simulink model "RR_grasping"  (R2020b)
settings: Solver=FixedStepAuto  StartTime=0  StopTime=10.0  FixedStep=0.001  MaxStep=0.05  RelTol=1e-3
values from neighbouring files (symbols this model uses):
  a0 = 0.99    [init.m]
  berta = 0.98    [init.m]
  csi = 1    [init.m]
  e_max = 0.05    [init.m]
  F_max = [2;2]    [init.m]
  F_weight = [0;-50]    [init.m]
  g = 9.81    [init.m]
  I1 = 1    [init.m]
  I2 = 1    [init.m]
  l1 = 1    [init.m]
  l2 = 1    [init.m]
  m1 = 1    [init.m]
  m2 = 1    [init.m]
  mass = 1    [init.m]
libraries: cstblocks x2, simulink x1
settings Model: Creator=chiara-s  LastModifiedBy=chiara-s

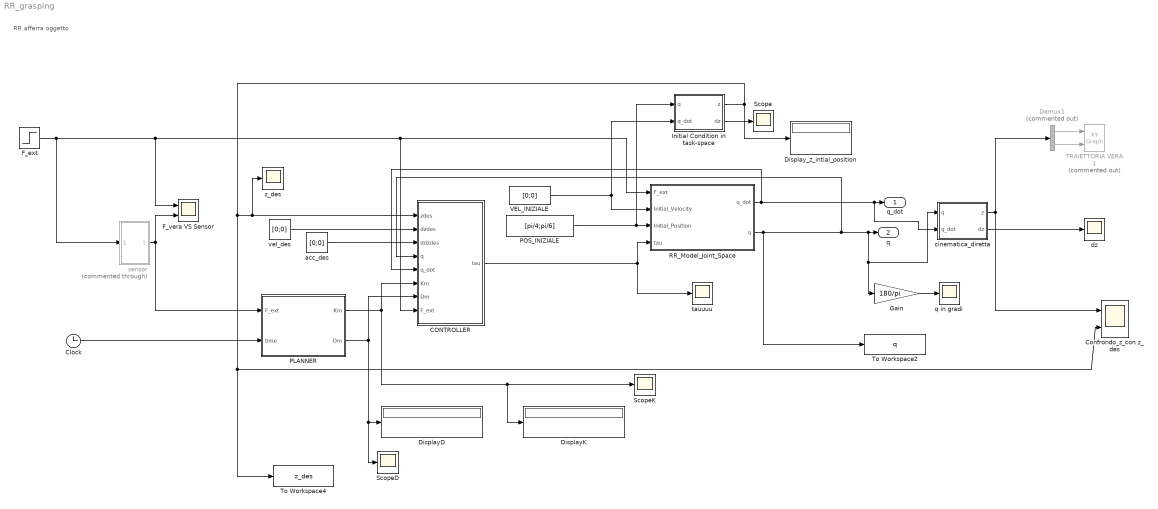
== system RR_grasping ==
  note: RR afferra oggetto
  CONTROLLER : MATLAB Function  TreatAsAtomicUnit=on
  Clock : Clock
  Confrondo_z_con z_des : Scope  NumInputPorts=2
  Demux1 : Demux  Commented=on  Outputs=2
  DisplayD : Display
  DisplayK : Display
  Display_z_intial_position : Display
  F_ext : Step  Before=[0;0]  After=2*F_weight  SampleTime=0
  F_vera VS Sensor : Scope  NumInputPorts=2
  Gain : Gain  Gain=180/pi
  Initial Condition in task-space : MATLAB Function  TreatAsAtomicUnit=on
  PLANNER : MATLAB Function  TreatAsAtomicUnit=on
  POS_INIZIALE : Constant  Value=[pi/4;pi/6]
  RR_Model_Joint_Space : Subsystem
  Scope : Scope
  ScopeD : Scope
  ScopeK : Scope
  TRAIETTORIA VERA 1 : simulink/Sinks/XY Graph  Commented=on  xmin=-2  xmax=2  ymin=-2  ymax=2  st=-1
  To Workspace2 : ToWorkspace  VariableName=q  SaveFormat=Structure With Time  SampleTime=-1
      settings: Save2DSignal=2-D array (concatenate along first dimension)
  To Workspace4 : ToWorkspace  VariableName=z_des  SaveFormat=Structure With Time  SampleTime=-1
      settings: Save2DSignal=2-D array (concatenate along first dimension)
  VEL_INIZIALE : Constant  Value=[0;0]
  acc_des : Constant  Value=[0;0]
  cinematica_diretta : MATLAB Function  TreatAsAtomicUnit=on
  dz : Scope
  q in gradi : Scope
  sensor : Subsystem  Commented=through
  tauuuu : Scope
  vel_des : Constant  Value=[0;0]
  z_des : Scope
  q_dot : Outport
  q : Outport  Port=2
  wires:
  RR_Model_Joint_Space/1(q_dot) -> cinematica_diretta/2(q_dot), q_dot/1, CONTROLLER/5(q_dot)
  Initial Condition in task-space/1(z) -> z_des/1, CONTROLLER/1(zdes), To Workspace4/1, Confrondo_z_con z_des/2, Display_z_intial_position/1
  F_ext/1 -> sensor/1(In1), RR_Model_Joint_Space/1(F_ext), CONTROLLER/8(F_ext), F_vera VS Sensor/1
  CONTROLLER/1(tau) -> tauuuu/1, RR_Model_Joint_Space/4(tau)
  PLANNER/1(Km) -> CONTROLLER/6(Km), ScopeK/1, DisplayK/1
  vel_des/1 -> CONTROLLER/2(dzdes)
  Demux1/2 -> TRAIETTORIA VERA 1/2
  PLANNER/2(Dm) -> CONTROLLER/7(Dm), ScopeD/1, DisplayD/1
  RR_Model_Joint_Space/2(q) -> CONTROLLER/4(q), Gain/1, cinematica_diretta/1(q), q/1, To Workspace2/1
  Demux1/1 -> TRAIETTORIA VERA 1/1
  cinematica_diretta/1(z) -> Confrondo_z_con z_des/1, Demux1/1
  cinematica_diretta/2(dz) -> dz/1
  POS_INIZIALE/1 -> RR_Model_Joint_Space/3(Initial_Position), Initial Condition in task-space/1(q)
  Gain/1 -> q in gradi/1
  VEL_INIZIALE/1 -> Initial Condition in task-space/2(q_dot), RR_Model_Joint_Space/2(Initial_Velocity)
  acc_des/1 -> CONTROLLER/3(ddzdes)
  Initial Condition in task-space/2(dz) -> Scope/1
  Clock/1 -> PLANNER/2(time)
  sensor/1(Out1) -> PLANNER/1(F_ext), F_vera VS Sensor/2

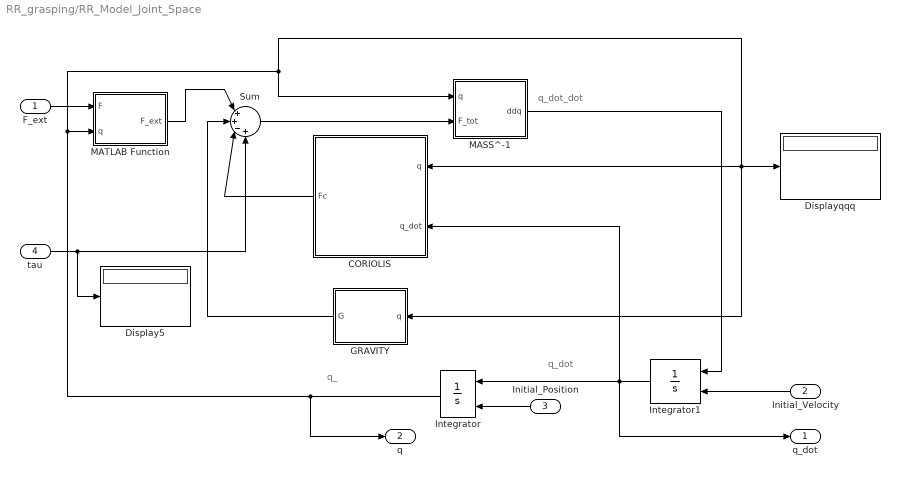
== system RR_grasping/RR_Model_Joint_Space ==
  note: q_dot
  note: q_dot_dot
  note: q_
  F_ext : Inport
  Initial_Velocity : Inport  Port=2
  Initial_Position : Inport  Port=3
  tau : Inport  Port=4
  CORIOLIS : MATLAB Function  TreatAsAtomicUnit=on
  Display5 : Display
  Displayqqq : Display
  GRAVITY : MATLAB Function  TreatAsAtomicUnit=on
  Integrator : Integrator  InitialConditionSource=external
  Integrator1 : Integrator  InitialConditionSource=external  InitialCondition=[0;0]
  MASS^-1 : MATLAB Function  TreatAsAtomicUnit=on
  MATLAB Function : MATLAB Function  TreatAsAtomicUnit=on
  Sum : Sum  Inputs=|++-+
  q_dot : Outport
  q : Outport  Port=2
  wires:
  GRAVITY/1(G) -> Sum/2
  MATLAB Function/1(F_ext) -> Sum/1
  Initial_Position/1 -> Integrator/2
  F_ext/1 -> MATLAB Function/1(F)
  Integrator/1 -> MASS^-1/1(q), GRAVITY/1(q), Displayqqq/1, CORIOLIS/1(q), MATLAB Function/2(q), q/1
  Integrator1/1 -> q_dot/1, CORIOLIS/2(q_dot), Integrator/1
  Initial_Velocity/1 -> Integrator1/2
  MASS^-1/1(ddq) -> Integrator1/1
  Sum/1 -> MASS^-1/2(F_tot)
  CORIOLIS/1(Fc) -> Sum/3
  tau/1 -> Display5/1, Sum/4

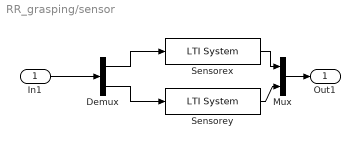
== system RR_grasping/sensor ==
  In1 : Inport
  Demux : Demux  Outputs=2
  Mux : Mux  Inputs=2
  Sensorex : cstblocks/LTI System  sys=tf(50^2,[1 0.3*2*50 50^2])  IC=[]
  Sensorey : cstblocks/LTI System  sys=tf(50^2,[1 0.3*2*50 50^2])  IC=[]
  Out1 : Outport
  wires:
  Demux/1 -> Sensorex/1
  Sensorex/1 -> Mux/1
  Sensorey/1 -> Mux/2
  Mux/1 -> Out1/1
  Demux/2 -> Sensorey/1
  In1/1 -> Demux/1

== matlab function RR_grasping/RR_Model_Joint_Space/MATLAB Function ==
  data: F input size=2; F_ext output double size=2; q input size=2; l1 parameter; l2 parameter
function F_ext = fcn(F,q,l1, l2)


Ja = [-l1*sin(q(1)) - l2*sin(q(1)+q(2)), -l2*sin(q(1)+q(2)); ...
    l1*cos(q(1)) + l2*cos(q(1)+q(2)), l2*cos(q(1)+q(2))];

F_ext = Ja'*F;

end

== matlab function RR_grasping/cinematica_diretta ==
  data: q input double size=2; q_dot input double size=2; z output double size=2; dz output double size=2; l1 parameter; l2 parameter
function [z,dz] = fcn(q,q_dot,l1, l2)

z = zeros(2,1);
z(1) = l1*cos(q(1)) + l2*cos(q(1)+q(2));
z(2) = l1*sin(q(1)) + l2*sin(q(1)+q(2));

Ja = zeros(2,2);
Ja = [-l1*sin(q(1)) - l2*sin(q(1)+q(2)), -l2*sin(q(1)+q(2)); ...
    l1*cos(q(1)) + l2*cos(q(1)+q(2)), l2*cos(q(1)+q(2))];

dz = zeros(2,1);
dz = Ja*q_dot;

end

== matlab function RR_grasping/CONTROLLER ==
  data: zdes input size=2; tau output double size=2; dzdes input size=2; ddzdes input size=2; q input size=2; q_dot input size=2; Km input; Dm input; F_ext input; M parameter
function tau = fcn(zdes, dzdes, ddzdes, q, q_dot, Km, Dm, F_ext, M)
%% PROBLEMA MATRICE DELLE MASSE NON DIAGONALE
coder.extrinsic('Jacobianoa','Jacobianoa_dot','Mass','Coriolis','Gravity','cin_dir')
dz = zeros(2,1);
z = zeros(2,1);
B = zeros(2,2);
S = zeros(2,2);
G = zeros(2,1);
Ja = zeros(2,2);
Ja_dot = zeros(2,2);
Bm = [M 0; 0 M];
Ja = Jacobianoa(q);
Ja_dot = Jacobianoa_dot(q,q_dot);

dz = Ja*q_dot;
z = cin_dir(q);

t = 0.1;
if (deg2rad(-0.1) < q(2)) && (q(2) < deg2rad(0.1)) || (deg2rad(179.9) < q(2)) && (q(2) < deg2rad(180.1)) || (deg2rad(-180.1) < q(2)) && (q(2) < deg2rad(-179.9))
    Ja_inv = (Ja')*inv(Ja*(Ja') + t^2*eye(2,2)); % Damp least square Jacobian method
else 
    Ja_inv = inv(Ja);
end

% Ja_inv = inv(Ja);

B = Mass(q);
Bx = (Ja_inv')* B * Ja_inv;
S = Coriolis(q,q_dot);
G = Gravity(q);
I = eye(2,2);
% tau = B * Ja_inv*(ddzdes - Ja_dot*q_dot) + ...
%     S*q_dot + (Ja')*(Dm*(dzdes - dz) + Km*(zdes- z)) + G;

tau = B*Ja_inv*(ddzdes - Ja_dot*q_dot + ...
    inv(Bm)*(Dm*(dzdes - dz) + Km*(zdes- z))) + S*q_dot - G + ...
    (Ja')*(Bx*inv(Bm) - I)*F_ext;

end

== matlab function RR_grasping/Initial Condition in task-space ==
  data: q input double size=2; q_dot input double size=2; z output double size=2; dz output double size=2; l1 parameter; l2 parameter
function [z,dz] = fcn(q,q_dot,l1, l2)

z = zeros(2,1);
z(1) = l1*cos(q(1)) + l2*cos(q(1)+q(2));
z(2) = l1*sin(q(1)) + l2*sin(q(1)+q(2));

Ja = zeros(2,2);
Ja = [-l1*sin(q(1)) - l2*sin(q(1)+q(2)), -l2*sin(q(1)+q(2)); ...
    l1*cos(q(1)) + l2*cos(q(1)+q(2)), l2*cos(q(1)+q(2))];

dz = zeros(2,1);
dz = Ja*q_dot;

end

== matlab function RR_grasping/PLANNER ==
  settings: updateMethod=DISCRETE
  data: Km output; Dm output; e_max parameter; F_max parameter; F_ext input; mass parameter; F_weight parameter; time input; a0 parameter; csi parameter; berta parameter
function [Km,Dm] = fcn(e_max, F_max, F_ext, mass, F_weight, time, a0, csi, berta)

% with an estimated weight, k and d increase 
%% Outputs
% Km            stiffness matrix
% Dm            damping matrix 
%% Inputs
% time          current simulation time
% F_ext         measured external force

% variables initialization 
persistent kx_i ky_i dx dy timeG kx ky F_grasp kx_f ky_f

if isempty(kx_f)
    kx_f = abs(F_weight(1))/e_max;
end

if isempty(ky_f)
    ky_f = abs(F_weight(2))/e_max;
end

if isempty(F_grasp)
    F_grasp = [0;0];
end

if isempty(timeG)
    timeG = 1000;
end

if isempty(kx)
   kx = abs(F_weight(1))/e_max; 
end
if isempty(ky)
   ky = abs(F_weight(2))/e_max;
end

% initialization of k and d 
if isempty(kx_i)
   kx_i = abs(F_weight(1))/e_max; 
end
if isempty(ky_i)
   ky_i = abs(F_weight(2))/e_max;
end
if isempty(dx)
    dx = sqrt(4*kx_i*mass);
end
if isempty(dy)
    dy = sqrt(4*ky_i*mass);
end

% definition of k_dot for stability condition (from article)
k_dotx = berta*(4*a0*sqrt(kx_i/mass)*(kx_i)^(3/2))/(sqrt(kx_i) + 2*a0*csi*sqrt(kx_i));
k_doty = berta*(4*a0*sqrt(ky_i/mass)*(ky_i)^(3/2))/(sqrt(ky_i) + 2*a0*csi*sqrt(ky_i));


% start algoritm with k variable
if abs(F_ext(1))/kx > e_max
    if timeG == 1000
        timeG = time;
    end
    kx_f = abs(F_ext(1))/e_max;
    % law for increasing k
    k_tempx = kx_i + k_dotx*(time -timeG);
    if k_tempx > kx_f
        kx = kx_f;
    else
        kx = k_tempx;
    end
    dx = sqrt(4*kx*mass);
    
end
if abs(F_ext(2))/ky > e_max
    if timeG == 1000
        timeG = time;
    end
    ky_f = abs(F_ext(2))/e_max;
    k_tempy = ky_i + k_doty*(time -timeG);
    if k_tempy > ky_f
        ky = ky_f;
    else
        ky = k_tempy;
    end
    dy = sqrt(4*ky*mass);
end

% set k istantaneously
% kx = abs(F_ext(1))/e_max;
% ky = abs(F_ext(2))/e_max;

% Final Values of D-K
Dm = diag([dx,dy]);
Km = diag([kx,ky]);

end

== matlab function RR_grasping/RR_Model_Joint_Space/CORIOLIS ==
  data: q input size=2; Fc output double size=2; q_dot input size=2; a parameter
function Fc = fcn(q,q_dot,a)

C = zeros(2,2);
C = [-a*sin(q(2))*q_dot(2), -a*sin(q(2))*q_dot(1)-a*sin(q(2)*q_dot(2)); ...
    a*sin(q(2))*q_dot(1), 0];

Fc = C*q_dot;

end

== matlab function RR_grasping/RR_Model_Joint_Space/GRAVITY ==
  data: q input size=2; G output double size=2; g parameter; l1 parameter; l2 parameter; m1 parameter; m2 parameter
function G = fcn(q,g, l1, l2, m1, m2)


G = [-(l1/2)*cos(q(1))*m1*g - m2*g*(l1*cos(q(1))+(l2/2)*cos(q(1)+q(2))); ...
    -m2*g*(l2/2)*cos(q(1)+q(2))];

end

== matlab function RR_grasping/RR_Model_Joint_Space/MASS^-1 ==
  data: q input size=2; ddq output size=2; F_tot input double size=2; I1 parameter; I2 parameter; l1 parameter; l2 parameter; m1 parameter; m2 parameter
function ddq = fcn(q,F_tot,I1, I2, l1, l2, m1, m2)


B = [((l1^2)/4)*m1 + I1 + m2*(l1^2) + m2*((l2^2)/4) + m2*l1*l2*cos(q(2)) + I2, m2*(((l1*l2)/2)*cos(q(2)) + (l2^2)/4) + I2; ...
    m2*(((l1*l2)/2)*cos(q(2)) + (l2^2)/4) + I2, m2*(l2^2)/4 + I2];


ddq = B\F_tot;                      % Ftot*M^-1

end
